simulink model "gt_LQR_control_example"  (R2021b)
settings: Solver=ode4  StartTime=0.0  StopTime=inf  FixedStep=0.1  RelTol=1e-3
undefined symbols (not defined in the file): Twist
libraries: robotlib x4
settings Model: Creator=user  LastModifiedBy=seunghwan
settings SolverCC: AlgebraicLoopSolver=TrustRegion
settings DebuggingCC: SFMachineParentedDataDiag=warning

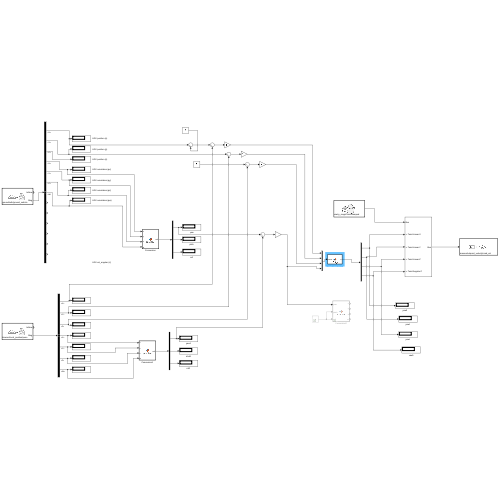
[thumbnail: Simulink's stored preview of the top-level diagram]
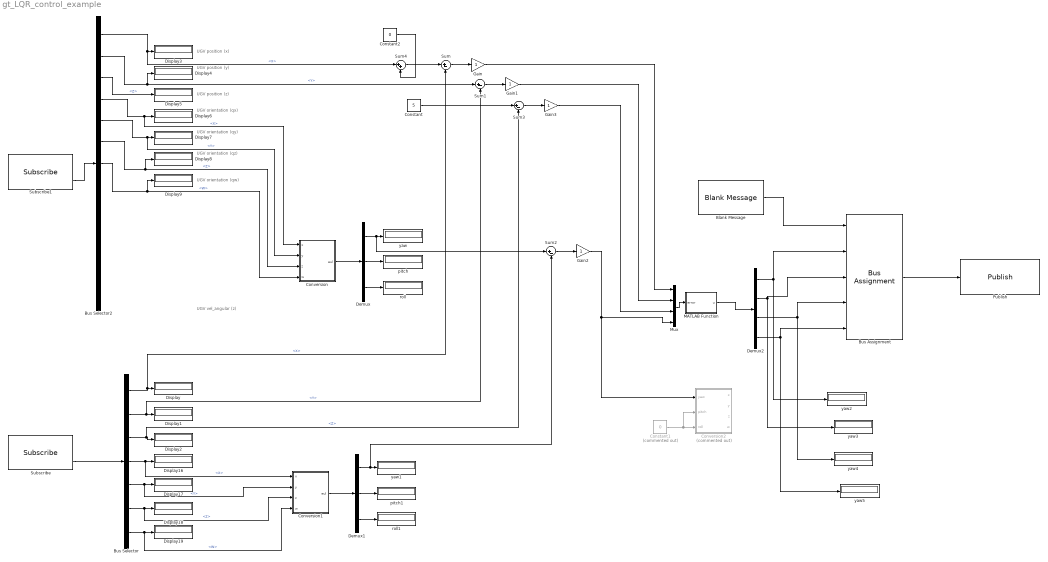
== system gt_LQR_control_example ==
  note: UGV position (x)
  note: UGV position (y)
  note: UGV position (z)
  note: UGV orientation (qx)
  note: UGV orientation (qy)
  note: UGV orientation (qz)
  note: UGV orientation (qw)
  note: UGV vel_angular (z)
  Blank Message : robotlib/Blank Message  messageClass=Message  entityType=geometry_msgs/TwistStamped  messageType=geometry_msgs/TwistStamped  SampleTime=0.1  legacyBusStruct=off
  Bus Assignment : BusAssignment  AssignedSignals=Twist.Linear.X,Twist.Linear.Y,Twist.Linear.Z,Twist.Angular.Z
  Bus Selector : BusSelector  OutputSignals=Pose.Position.X,Pose.Position.Y,Pose.Position.Z,Pose.Orientation.X,Pose.Orientation.Y,Pose.Orientation.Z,Pose.Orientation.W
  Bus Selector2 : BusSelector  OutputSignals=Pose.Pose.Position.X,Pose.Pose.Position.Y,Pose.Pose.Position.Z,Pose.Pose.Orientation.X,Pose.Pose.Orientation.Y,Pose.Pose.Orientation.Z,Pose.Pose.Orientation.W,Twist.Twist.Linear.X,Twist.Twist.Linear.Y,Twist.Twist.Linear.Z,Twist.Twist.Angular.X,Twist.Twist.Angular.Y,Twist.Twist.Angular.Z
  Constant : Constant  Value=5
  Constant1 : Constant  Commented=on  Value=0
  Constant2 : Constant  Value=0
  Conversion : MATLAB Function  TreatAsAtomicUnit=on
  Conversion1 : MATLAB Function  TreatAsAtomicUnit=on
  Conversion2 : MATLAB Function  Commented=on  TreatAsAtomicUnit=on
  Demux : Demux  Outputs=3
  Demux1 : Demux  Outputs=3
  Demux2 : Demux
  Display{,1..9,16..19} (14 alike) : Display
  Gain{,1..3} (4 alike) : Gain
  MATLAB Function : MATLAB Function  TreatAsAtomicUnit=on
  Mux : Mux
  Publish : robotlib/Publish  topicSource=Select from ROS network  topic=/mavros/setpoint_velocity/cmd_vel  messageType=geometry_msgs/TwistStamped  legacyBusStruct=off  messageQueueLength=1
  Subscribe : robotlib/Subscribe  topicSource=Select from ROS network  topic=/mavros/local_position/pose  messageType=geometry_msgs/PoseStamped  SampleTime=-1  legacyBusStruct=off  messageQueueLength=1
  Subscribe1 : robotlib/Subscribe  topicSource=Select from ROS network  topic=/gazebo_groundtruth/ground_vehicle  messageType=nav_msgs/Odometry  SampleTime=-1  legacyBusStruct=off  messageQueueLength=1
  Sum{,1..3} (4 alike) : Sum  Inputs=|+-
  Sum4 : Sum  Inputs=|++
  pitch : Display
  pitch1 : Display
  roll : Display
  roll1 : Display
  yaw{,1..5} (6 alike) : Display
  wires:
  Bus Selector/1 -> Display/1, Sum/2  "<X>"
  Bus Selector/3 -> Sum3/2, Display2/1  "<Z>"
  Blank Message/1 -> Bus Assignment/1
  Bus Assignment/1 -> Publish/1
  Subscribe1/2 -> Bus Selector2/1
  Bus Selector2/4 -> Conversion/1(x), Display6/1  "<X>"
  Bus Selector2/5 -> Conversion/2(y), Display7/1  "<Y>"
  Bus Selector2/6 -> Display8/1, Conversion/3(z)  "<Z>"
  Bus Selector2/7 -> Display9/1, Conversion/4(w)  "<W>"
  Sum/1 -> Gain/1
  Sum1/1 -> Gain1/1
  Bus Selector/2 -> Sum1/2, Display1/1  "<Y>"
  Demux/2 -> pitch/1
  Demux/3 -> roll/1
  Conversion/1(eul) -> Demux/1
  Demux/1 -> Sum2/1, yaw/1
  Constant1/1 -> Conversion2/2(pitch), Conversion2/3(roll)
  Sum2/1 -> Gain2/1
  Gain2/1 -> Mux/4, Conversion2/1(yaw)
  Gain1/1 -> Mux/2
  Gain/1 -> Mux/1
  Sum3/1 -> Gain3/1
  Demux1/1 -> Sum2/2, yaw1/1
  Conversion1/1(eul) -> Demux1/1
  Demux1/3 -> roll1/1
  Demux1/2 -> pitch1/1
  Bus Selector/4 -> Conversion1/1(x), Display16/1  "<X>"
  Bus Selector/5 -> Conversion1/2(y), Display17/1  "<Y>"
  Bus Selector/6 -> Conversion1/3(z), Display18/1  "<Z>"
  Bus Selector/7 -> Conversion1/4(w), Display19/1  "<W>"
  Gain3/1 -> Mux/3
  Subscribe/2 -> Bus Selector/1
  Constant/1 -> Sum3/1
  Demux2/1 -> yaw2/1, Bus Assignment/2
  Demux2/2 -> yaw3/1, Bus Assignment/3
  Demux2/3 -> yaw4/1, Bus Assignment/4
  Demux2/4 -> yaw5/1, Bus Assignment/5
  Mux/1 -> MATLAB Function/1(error)
  MATLAB Function/1(u) -> Demux2/1
  Bus Selector2/1 -> Sum4/1, Display3/1  "<X>"
  Bus Selector2/2 -> Display4/1, Sum1/1  "<Y>"
  Bus Selector2/3 -> Display5/1  "<Z>"
  Constant2/1 -> Sum4/2
  Sum4/1 -> Sum/1

== matlab function gt_LQR_control_example/Conversion1 ==
  data: eul output; x input; y input; z input; w input
function eul  = quat2eul(x,y,z,w)
%#codegen

% Convert the quaternion to a yaw angle (zyx euler angle)
eul = quat2eul([w,x,y,z]);
% yaw = eul(1);

end

== matlab function gt_LQR_control_example/Conversion ==
  data: eul output; x input; y input; z input; w input
function eul  = quat2eul(x,y,z,w)
%#codegen

% Convert the quaternion to a yaw angle (zyx euler angle)
eul = quat2eul([w,x,y,z]);
% yaw = eul(1);

end

== matlab function gt_LQR_control_example/Conversion2 ==
  data: yaw input; pitch input; roll input; x output; y output; z output; w output
function [x,   y,   z,   w]   = eul2quat(yaw,pitch,roll)
%#codegen

% Convert the quaternion to a yaw angle (zyx euler angle)
q = eul2quat([yaw,pitch,roll]);
w=q(1);
x=q(2);
y=q(3);
z=q(4);
end

== matlab function gt_LQR_control_example/MATLAB Function ==
  data: error input; u output
function u=LQR_K(error)
coder.extrinsic('lqr');
n=length(error);
dt=1.5;
N=zeros(n);
A=eye(n);
B=dt*eye(n);
Q=eye(n);
R=eye(n);
Q(1,1)=10;
Q(3,3)=0.01;
K=zeros(n);

[K, S, e]=lqr(A,B,Q,R,N);

u=K*error;
